simulink model "experiment_6_b"  (R2018b)
settings: Solver=VariableStepAuto  StartTime=0.0  StopTime=0.1  RelTol=1e-3
libraries: commsrccod2 x2, simulink x2
settings Model: Creator=sangh  LastModifiedBy=sangh

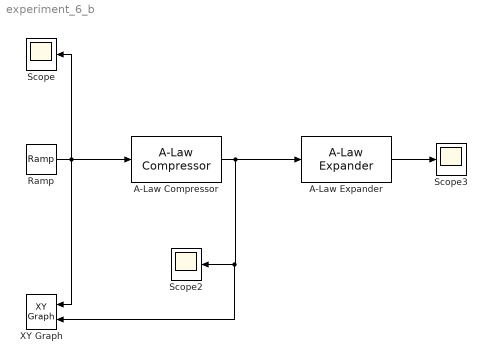
== system experiment_6_b ==
  A-Law Compressor : commsrccod2/A-Law Compressor  A=87.6  V=1
      settings: SourceProductName=Communications System Toolbox  SourceProductBaseCode=CM
  A-Law Expander : commsrccod2/A-Law Expander  A=87.6  V=1
      settings: SourceProductName=Communications System Toolbox  SourceProductBaseCode=CM
  Ramp : simulink/Sources/Ramp  slope=20  start=0  InitialOutput=-1
  Scope : Scope
  Scope2 : Scope
  Scope3 : Scope
  XY Graph : simulink/Sinks/XY Graph  xmin=-1  xmax=1  ymin=-1  ymax=1  st=-1
  wires:
  Ramp/1 -> XY Graph/1, A-Law Compressor/1, Scope/1
  A-Law Compressor/1 -> A-Law Expander/1, XY Graph/2, Scope2/1
  A-Law Expander/1 -> Scope3/1
